simulink model "mavsim_chap10_6DOF"  (R2020b)
settings: Solver=ode15s  StartTime=0.0  StopTime=400  RelTol=1e-3  EnableMultiTasking=on
InitFcn:
  | param_chap10
undefined symbols (not defined in the file or in its folder): autopilot, drawPathError, Earth, forces_moments, js_decode_landing, js_encode_landing, P, path_follow, path_manager_chap10, sigbuilder_block, true_states, WGS84
libraries: simulink x7, simulink_extras x7, pid_lib x7, aerolibfltsims x2, instrumentlib x2, shared6dof x1, aerolibasang x1, aerolibtransform2 x1, aerolibanimutils x1, dspnetwork x1
(part 2 of 2)

== system mavsim_chap10_6DOF/Subsystem5/Controlled MAV/Wind1 ==
  Constant1 : Constant  Value=[0; 0; 0]
  Constant2 : Constant  Value=[P.wind_n; P.wind_e; P.wind_d]
  Mux1 : Mux  Inputs=2
  Wind Gusts : Subsystem
  Wind : Outport
  wires:
  Constant2/1 -> Mux1/1
  Mux1/1 -> Wind/1
  Constant1/1 -> Mux1/2

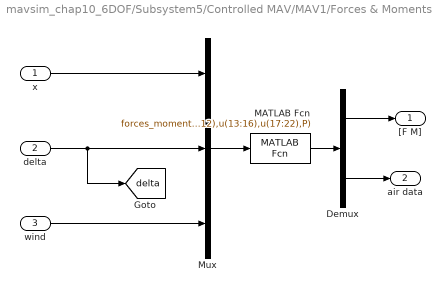
== system mavsim_chap10_6DOF/Subsystem5/Controlled MAV/MAV1/Forces & Moments ==
  x : Inport
  delta : Inport  Port=2
  wind : Inport  Port=3
  Demux : Demux  Outputs=[6;6]
  MATLAB Fcn : MATLABFcn  MATLABFcn=forces_moments(u(1:12),u(13:16),u(17:22),P)  OutputDimensions=12
  Mux : Mux  Inputs=3
  "[F M]" : Outport
  air data : Outport  Port=2
  tag scope: delta=global
  wires:
  x/1 -> Mux/1
  delta/1 -> [delta], Mux/2
  wind/1 -> Mux/3
  MATLAB Fcn/1 -> Demux/1
  Demux/1 -> "[F M]"/1
  Mux/1 -> MATLAB Fcn/1
  Demux/2 -> air data/1

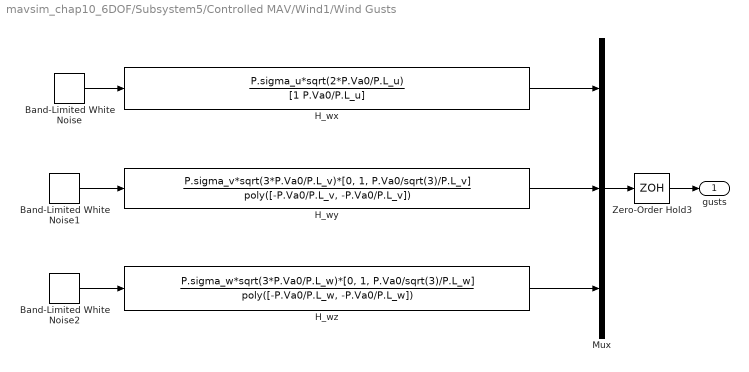
== system mavsim_chap10_6DOF/Subsystem5/Controlled MAV/Wind1/Wind Gusts ==
  Band-Limited White Noise : simulink/Sources/Band-Limited White Noise  Cov=[1]  Ts=P.Ts  seed=[23341]
  Band-Limited White Noise1 : simulink/Sources/Band-Limited White Noise  Cov=[1]  Ts=P.Ts  seed=[23341]
  Band-Limited White Noise2 : simulink/Sources/Band-Limited White Noise  Cov=[1]  Ts=P.Ts  seed=[23341]
  H_wx : TransferFcn  Numerator=P.sigma_u*sqrt(2*P.Va0/P.L_u)  Denominator=[1 P.Va0/P.L_u]
  H_wy : TransferFcn  Numerator=P.sigma_v*sqrt(3*P.Va0/P.L_v)*[0, 1, P.Va0/sqrt(3)/P.L_v]  Denominator=poly([-P.Va0/P.L_v, -P.Va0/P.L_v])
  H_wz : TransferFcn  Numerator=P.sigma_w*sqrt(3*P.Va0/P.L_w)*[0, 1, P.Va0/sqrt(3)/P.L_w]  Denominator=poly([-P.Va0/P.L_w, -P.Va0/P.L_w])
  Mux : Mux  Inputs=3
  Zero-Order Hold3 : ZeroOrderHold  SampleTime=P.Ts
  gusts : Outport
  wires:
  Zero-Order Hold3/1 -> gusts/1
  Mux/1 -> Zero-Order Hold3/1
  Band-Limited White Noise2/1 -> H_wz/1
  H_wz/1 -> Mux/3
  Band-Limited White Noise1/1 -> H_wy/1
  H_wy/1 -> Mux/2
  Band-Limited White Noise/1 -> H_wx/1
  H_wx/1 -> Mux/1

== matlab function mavsim_chap10_6DOF/LandingGear ==
  data: z input; Fe output; Vz input
function Fe = fcn(z,Vz)
h = -z;
Vh = -Vz;
c = 300000*4;
d = 100000*4;
contact = h < 0;
if contact
    fc = -c*abs(h);
    fd2 = d*Vh;
else
    fc = 0;
    fd2 = 0;
end
if contact
    if fd2 < fc 
        fd = fc;
    elseif fd2 > -fc
        fd = -fc;
    else
        fd = fd2;
    end
else
    fd = 0;
end
Fe = zeros(3,1);
Fe(1) = 0;
Fe(2) = 0;
Fe(3) = fc + fd;

== matlab function mavsim_chap10_6DOF/Force Moment ==
  data: alpha input; beta input; da input; de input; dr input; T input; F output; V input; p_B input; M output; q_B input; r_B input; t input; time input; z input
function [F,M] = fcn(alpha,beta,da,de,dr,T,V,p_B,q_B,r_B,t,time,z)
cbar=10;
lt=10;
St=5;
S=20;
rho=1.22505;
V_A = norm(V);
q_dyn=rho/2.0*V_A*V_A;
qS=q_dyn*S;
cLwb_alpha=3.5;
alpha0=5*pi/180;
cLwb=cLwb_alpha*(alpha + alpha0);
cLt_alpha=1.5;
epps=0.25*(alpha + alpha0);
alpha_tail=alpha - epps+ de + 1.3*q_B*lt/V_A;
cLt=cLt_alpha*alpha_tail*St/S;
cL=cLwb+cLt;
cD_0=0.03;
cD_cL_min=0.15;
cD_cL2=0.07;
cD=cD_0+cD_cL2*(cLwb-cD_cL_min)^2;
cY_beta=-1.6;
cY_rudder=0.24;
cY=cY_beta*beta+cY_rudder*dr;
Tbs=[cos(alpha)*cos(beta),-cos(alpha)*sin(beta),-sin(alpha);...
     sin(beta),            cos(beta),          0;...
     sin(alpha)*cos(beta),-sin(alpha)*sin(beta),cos(alpha)];
F_S=qS.*[-cD;cY;-cL];
F_B=Tbs*F_S+[T;0;0];
if time >= t 
    if V(1) >= 1e-8 && z >=-1 
        F_brake = -11000*27; 
    else
        F_brake = 0;
    end
else
    F_brake = 0;
end
F = zeros(3,1);  
if z <= -100
    F(1)=F_B(1) - 11000*2
else
    F(1)=F_B(1) + F_brake;
end
F(2)=F_B(2);
F(3)=F_B(3);
cl_beta=-1.4;
cm_0=-0.59;
cn_beta=1;
cn_alphabeta=-1/15.0*180/pi;
clmn0=[cl_beta*beta;    cm_0 - cLt*lt/cbar;     cn_beta*beta + cn_alphabeta*alpha*beta];
clmnRot=[-11.0,     0,    5.0;...
         0,    -5,      0;...
         1.7,     0,  -11.5];
clmnAct=[ -0.6,     0,   0.22;...
         0,   -10,      0;...
         0,     0,  -0.63];
clmn=clmn0+clmnRot*[p_B;q_B;r_B]*cbar/V_A+clmnAct*[da;de;dr];
M_B=qS*cbar*clmn;
M = zeros(3,1);
M(1)=M_B(1);
M(2)=M_B(2);
M(3)=M_B(3);

end

== matlab function mavsim_chap10_6DOF/MATLAB Function1 ==
  data: u input; y output; time input
function y = fcn(u,time)
if u < 1 
    y = u;
else
    if time < u+2
        y = 0;
    else
        y = u+2;
    end
end

== matlab function mavsim_chap10_6DOF/MATLAB Function ==
  data: u input; u1 input; u2 input; u3 input; y output; time input
function y = fcn(u,u1,u2,u3,time)
if u<=0
    y = -600;
else
    if time < u+2
        y = -600;
    else
        y = (time-u-2)*(-290+600)/(50-3)-600; 
    end
    if u1 <= 0
    else
        if time > u1+2
            y = (u1+2-u-2)*(-290+600)/(50-3)-600;
        end
    end
    if u2 <= 0
    else
        if time > u2+2
            y_ini = (u1+2-u-2)*(-290+600)/(50-3)-600;
            y = (time-u2-2)*(-290+600)/(50-3)+y_ini;
        end
    end
    if u3 <=0
    else
        if time > u3+2
            y1_ini = (u1+2-u-2)*(-290+600)/(50-3)-600;
            y2_ini = y1_ini;
            y3_ini = (u3+2-u2-2)*(-290+600)/(50-3)+y2_ini;
            y = (time-u3-2)*290/(64-50)+y3_ini;
        end
    end 
    if y >= 0
        y = 0;
    end
end

end

== matlab function mavsim_chap10_6DOF/MATLAB Function2 ==
  data: y output uint8; u1 input; u2 input
function  y = json_encode(u1,u2)
S = struct("StartLanding",...
            struct("id", 1,"type","int","data", u1,"dirction","IN","info","ToMatlab,0_NotAllowed,1_Allowed"),...
            "Landing",....
            struct("id", 2,"type","int","data", u2,"dirction","IN","info","ToMatlab,0_null,1_start"),...
            "LandingDeviation",....
            struct("id", 3,"type","data","data", [1,2,3],"dirction","IN","info","ToMatlab,Landing Deviation Information"),...
            "ReFly",....
            struct("id", 4,"type","int","data", 0,"dirction","IN","info","ToMatlab,ReFly Information"));
coder.extrinsic('jsonencode');
result = jsonencode(S);
y = uint8(zeros(1,406));
y =  uint8(result);

== matlab function mavsim_chap10_6DOF/jiaban1/MATLAB Function2 ==
  data: u input; y output; t input
function y = fcn(u,t)
if u <= 0
    start_time = 0;
    y = 0;
else
    start_time = u;
    y = (t-start_time)*15;
end

== matlab function mavsim_chap10_6DOF/jiaban2/MATLAB Function2 ==
  data: u input; y output; t input
function y = fcn(u,t)
if u <= 0
    start_time = 0;
    y = 0;
else
    start_time = u;
    y = (t-start_time)*4;
end

== matlab function mavsim_chap10_6DOF/MATLAB Function3 ==
  data: u input; y output; u1 input
function y = fcn(u,u1)
if u
    if u1
        y = 0;
    else
        y = 1;
    end
else
    y = 0;
end
